simulink model "linear_ss_control_reg"  (R2019b)
settings: Solver=ode45  StartTime=0.0  StopTime=1500  MaxStep=0.01  RelTol=1e-8
settings Model: Creator=Hector  LastModifiedBy=Hector

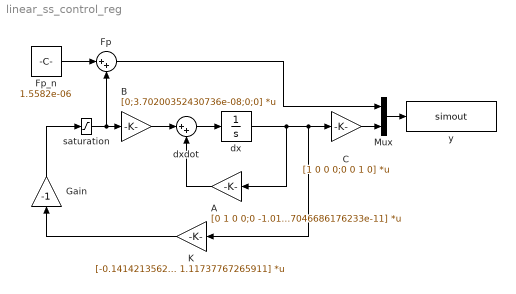
== system linear_ss_control_reg ==
  A : Gain  Gain=[0 1 0 0;0 -1.01409337235247e-10 -1.70834505909243e-20 -3.36920663455173e-10;0 0 0 1;0 15365.0510962495 3.88260240702825e-06 -5.07046686176233e-11]  Multiplication=Matrix(K*u)
  B : Gain  Gain=[0;3.70200352430736e-08;0;0]  Multiplication=Matrix(K*u)
  C : Gain  Gain=[1 0 0 0;0 0 1 0]  Multiplication=Matrix(K*u)
  Fp : Sum  Inputs=|++
  Fp_n : Constant  Value=1.5582e-06
  Gain : Gain  Gain=-1
  K : Gain  Gain=[-0.141421356249834 963078.733398081 0.010243364845765 1.11737767265911]  Multiplication=Matrix(K*u)
  Mux : Mux  Inputs=2
  dx : Integrator  InitialCondition=[0, 0, -1*10^-3, 0].'
  dxdot : Sum  Inputs=|++
  saturation : Saturate  UpperLimit=1.8442e-05  LowerLimit=-1.5582e-06
  y : ToWorkspace  VariableName=simout  SaveFormat=Timeseries  SampleTime=-1
  wires:
  dxdot/1 -> dx/1
  A/1 -> dxdot/2
  dx/1 -> C/1, K/1, A/1
  B/1 -> dxdot/1
  K/1 -> Gain/1
  Fp_n/1 -> Fp/1
  Gain/1 -> saturation/1
  Mux/1 -> y/1
  C/1 -> Mux/2
  Fp/1 -> Mux/1
  saturation/1 -> B/1, Fp/2
